simulink model "Linearized_controller"  (R2017b)
settings: Solver=VariableStepAuto  StartTime=0.0  StopTime=10.0  RelTol=1e-3
settings Model: Creator=Jesus  LastModifiedBy=Jesus

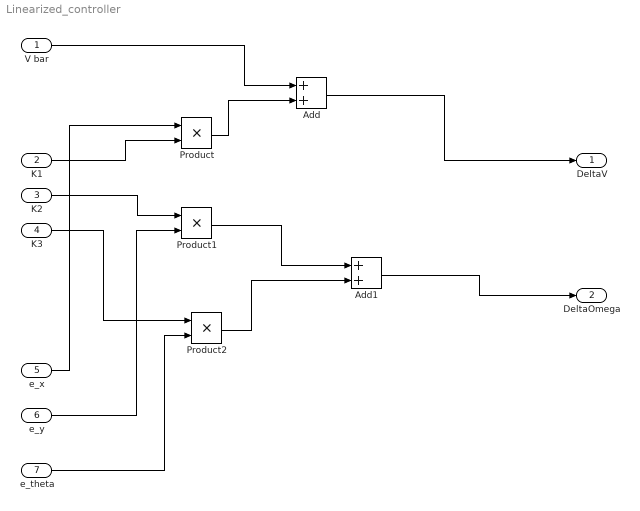
== system Linearized_controller ==
  "V bar " : Inport
  "K1 " : Inport  Port=2
  "K2 " : Inport  Port=3
  "K3 " : Inport  Port=4
  "e_x " : Inport  Port=5
  "e_y " : Inport  Port=6
  "e_theta " : Inport  Port=7
  Add : Sum
  Add1 : Sum
  Product : Product
  Product1 : Product
  Product2 : Product
  DeltaV : Outport
  "DeltaOmega " : Outport  Port=2
  wires:
  "V bar "/1 -> Add/1
  "e_x "/1 -> Product/1
  "K1 "/1 -> Product/2
  Product/1 -> Add/2
  Add/1 -> DeltaV/1
  "K2 "/1 -> Product1/1
  "e_y "/1 -> Product1/2
  Product1/1 -> Add1/1
  "K3 "/1 -> Product2/1
  "e_theta "/1 -> Product2/2
  Product2/1 -> Add1/2
  Add1/1 -> "DeltaOmega "/1
